simulink model "auv_nmpc_cbf"  (R2024a)
settings: Solver=ode4  StartTime=0.0  StopTime=35  FixedStep=0.010  RelTol=1e-3
values from neighbouring files (symbols this model uses):
  cbfParms = testValues(i,:)    [sweep_auv_cbf.m]
  obstacle = [obs_x , obs_y, obs_z, thisObsRadius]    [sweep_auv_cbf.m]
libraries: simulink x4
settings Model: Creator=mpent  LastModifiedBy=14244039
settings DebuggingCC: UnconnectedInputMsg=warning  UnconnectedOutputMsg=warning  UnconnectedLineMsg=warning
settings ModelReferenceCC: EnableRefExpFcnMdlSchedulingChecks=on
settings RTWCC: GPUComputeCapability=3.5  DLArmComputeVersion=19.05

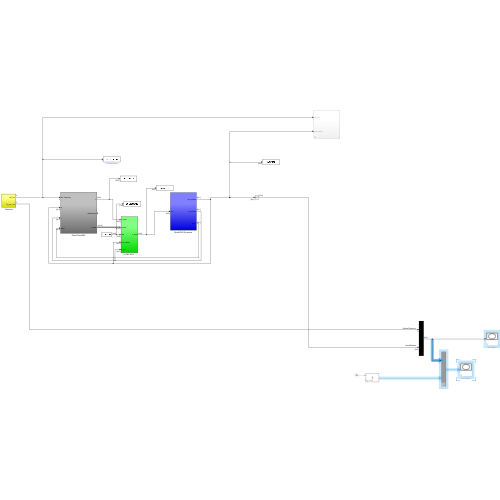
[thumbnail: Simulink's stored preview of the top-level diagram]
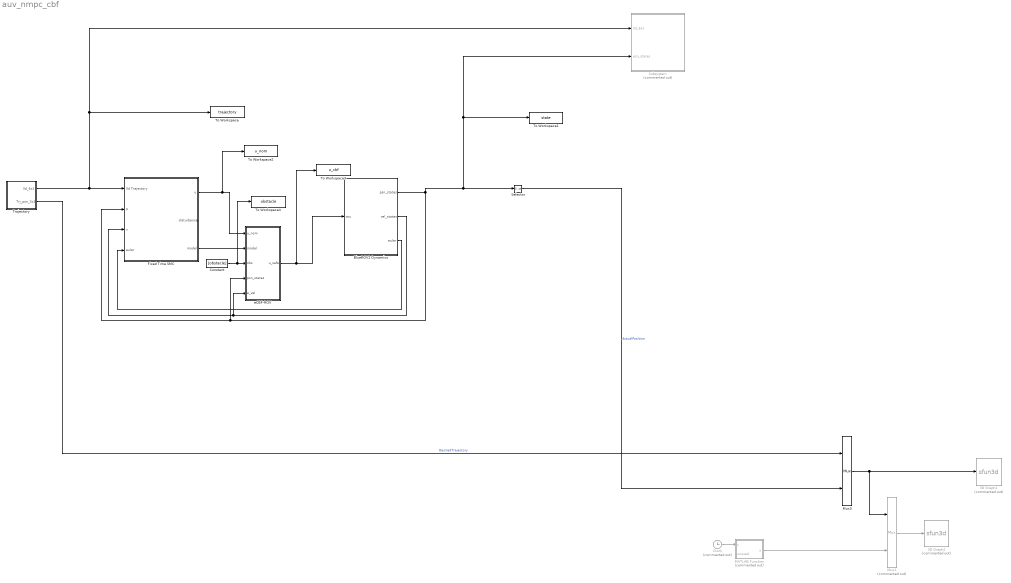
== system auv_nmpc_cbf ==
  3D Graph1 : S-Function  Commented=on  LoadFcn=if exist('sfun3d','file'), sfun3d([],[],[],'LoadBlock'); end  FunctionName=sfun3d  Parameters=ax,T,np,cp,gd,ls,mk,mx,hd,tb  SFunctionDeploymentMode=off  EnableBusSupport=off  mask(3D Graph){np=2, ax=[1 11 1 11 1 11], mx=1e4, T=-1, cp=[180 45 90], gd=on, hd=on, tb=on, ls=-, mk=none}
      mask prompts: np "Number of moving points (lines)"; ax "Range: [xmin xmax  ymin ymax zmin zmax]"; mx "Max number of points in each line"; T "Sampling Time"; cp "Camera position (use [0 0 1] for 2D XY view)"; gd "Grid (on|off)"; hd "HeadMarkers (on|off)"; tb "Toolbar (on|off)"; ls "LineStyle"; mk "LineMarker"
      mask help:
      | This block plots the position of several points in the XYZ space. The input contains the coordinates of all the points (x1,y1,z1,x2,y2,z2,...).
      | The number of moving points (lines), the XYZ ranges, sampling time, camera position, and grid (among other things) can be set as mask parameters.
      settings: CopyFcn=if exist('sfun3d','file'), sfun3d([],[],[],'CopyBlock'); end  DeleteFcn=if exist('sfun3d','file'), sfun3d([],[],[],'DeleteBlock'); end  NameChangeFcn=if exist('sfun3d','file'), sfun3d([],[],[],'NameChange'); end
      mask Help:
      | This block plots the position of several points in the XYZ space. The input contains the coordinates of all the points (x1,y1,z1,x2,y2,z2,...).
      | The number of moving points (lines), the XYZ ranges, sampling time, camera position, and grid (among other things) can be set as mask parameters.
      mask TypeOptions ls: - | -- | : | -. | none
      mask TypeOptions mk: none | . | + | o | * | x | square | diamond | v | ^ | > | < | pentagram | hexagram
      mask Display: plot([.05 .95 .95 .05 .05],[.45 .45 .95 .95 .45], 0.5+cos(0:0.1:2*pi)*0.3,0.7+sin(0:0.1:2*pi)*0.2)
  3D Graph2 : S-Function  Commented=on  LoadFcn=if exist('sfun3d','file'), sfun3d([],[],[],'LoadBlock'); end  FunctionName=sfun3d  Parameters=ax,T,np,cp,gd,ls,mk,mx,hd,tb  SFunctionDeploymentMode=off  EnableBusSupport=off  mask(3D Graph){np=5, ax=[1 11 1 11 1 11], mx=1e4, T=-1, cp=[68.5220  -51.3281   23.4494], gd=on, hd=off, tb=on, ls=-, mk=none}
      mask prompts: np "Number of moving points (lines)"; ax "Range: [xmin xmax  ymin ymax zmin zmax]"; mx "Max number of points in each line"; T "Sampling Time"; cp "Camera position (use [0 0 1] for 2D XY view)"; gd "Grid (on|off)"; hd "HeadMarkers (on|off)"; tb "Toolbar (on|off)"; ls "LineStyle"; mk "LineMarker"
      mask help:
      | This block plots the position of several points in the XYZ space. The input contains the coordinates of all the points (x1,y1,z1,x2,y2,z2,...).
      | The number of moving points (lines), the XYZ ranges, sampling time, camera position, and grid (among other things) can be set as mask parameters.
      settings: CopyFcn=if exist('sfun3d','file'), sfun3d([],[],[],'CopyBlock'); end  DeleteFcn=if exist('sfun3d','file'), sfun3d([],[],[],'DeleteBlock'); end  NameChangeFcn=if exist('sfun3d','file'), sfun3d([],[],[],'NameChange'); end
      mask Help:
      | This block plots the position of several points in the XYZ space. The input contains the coordinates of all the points (x1,y1,z1,x2,y2,z2,...).
      | The number of moving points (lines), the XYZ ranges, sampling time, camera position, and grid (among other things) can be set as mask parameters.
      mask TypeOptions ls: - | -- | : | -. | none
      mask TypeOptions mk: none | . | + | o | * | x | square | diamond | v | ^ | > | < | pentagram | hexagram
      mask Display: plot([.05 .95 .95 .05 .05],[.45 .45 .95 .95 .45], 0.5+cos(0:0.1:2*pi)*0.3,0.7+sin(0:0.1:2*pi)*0.2)
  BlueROV2 Dynamics : Subsystem
  Clock : Clock  Commented=on
  Constant : Constant  Value=[obstacle]  VectorParams1D=off
  Fixed Time SMC : Subsystem
  MATLAB Function : MATLAB Function  Commented=on  TreatAsAtomicUnit=on
  Mux1 : Mux  Commented=on  Inputs=2
  Mux3 : Mux  Inputs=2
  Selector : Selector  InputPortWidth=6  IndexOptions=Index vector (dialog)  Indices=1:3  OutputSizes=1
  Subsystem : Subsystem  Commented=on
  To Workspace : ToWorkspace  VariableName=trajectory  SaveFormat=Timeseries  SampleTime=-1
  To Workspace1 : ToWorkspace  VariableName=state  SaveFormat=Timeseries  SampleTime=-1
  To Workspace2 : ToWorkspace  VariableName=u_nom  SaveFormat=Timeseries  SampleTime=-1
  To Workspace3 : ToWorkspace  VariableName=u_cbf  SaveFormat=Timeseries  SampleTime=-1
  To Workspace4 : ToWorkspace  VariableName=obstacle  SampleTime=-1
      settings: MaxDataPoints=1
  Trajectory : Subsystem
  eCBF-ROV : Subsystem
  wires:
  Mux3/1 -> Mux1/1, 3D Graph1/1
  Selector/1 -> Mux3/2  "ActualPosition"
  Trajectory/2(Trj_psn_3x1) -> Mux3/1  "DesiredTrajectory"
  BlueROV2 Dynamics/2(vel_states) -> Fixed Time SMC/3(v), eCBF-ROV/5(e_vel)
  BlueROV2 Dynamics/1(psn_states) -> To Workspace1/1, Subsystem/2(psn_states), Selector/1, eCBF-ROV/4(psn_states), Fixed Time SMC/2(p)
  BlueROV2 Dynamics/3(euler) -> Fixed Time SMC/4(euler)
  Trajectory/1(Xd_6x1) -> To Workspace/1, Subsystem/1(Xd_6x1), Fixed Time SMC/1(Xd Trajectory)
  Fixed Time SMC/1(u) -> To Workspace2/1, eCBF-ROV/1(u_nom)
  Constant/1 -> To Workspace4/1, eCBF-ROV/3(obs)
  Fixed Time SMC/3(model) -> eCBF-ROV/2(model)
  eCBF-ROV/1(u_safe) -> To Workspace3/1, BlueROV2 Dynamics/1(tau)
  Clock/1 -> MATLAB Function/1(t)
  MATLAB Function/1(y) -> Mux1/2
  Mux1/1 -> 3D Graph2/1

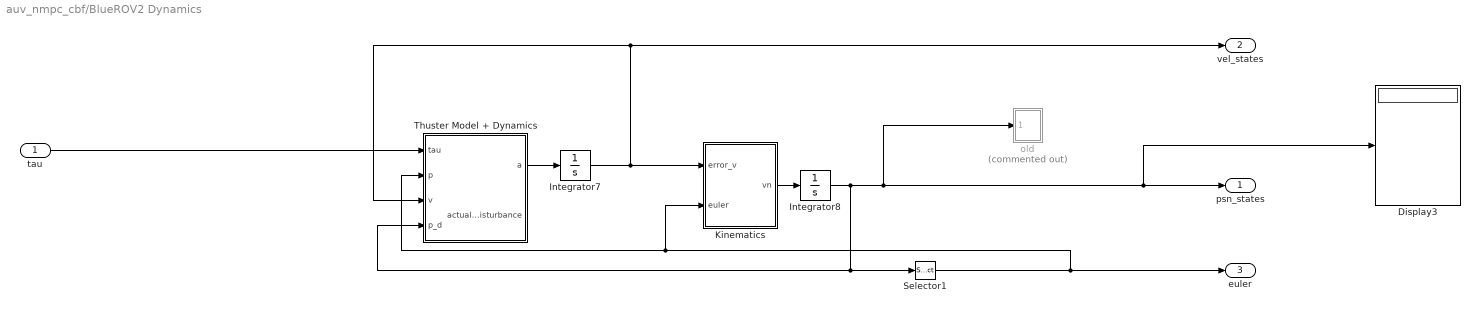
== system auv_nmpc_cbf/BlueROV2 Dynamics ==
  tau : Inport
  Display3 : Display
  Integrator7 : Integrator  InitialCondition=[0 0 0 0 0 0]'  LimitOutput=on  UpperSaturationLimit=[1 1 1 1 1 1]'*2  LowerSaturationLimit=[-1 -1 -1 -1 -1 -1]'*2
  Integrator8 : Integrator  InitialCondition=[1 1 1 0 0 0]'
  Kinematics : MATLAB Function  TreatAsAtomicUnit=on
  Selector1 : Selector  InputPortWidth=6  IndexOptions=Index vector (dialog)  Indices=4:6  OutputSizes=1
  Thuster Model + Dynamics : MATLAB Function  TreatAsAtomicUnit=on
  old : Subsystem  Commented=on
  psn_states : Outport
  vel_states : Outport  Port=2
  euler : Outport  Port=3
  wires:
  Selector1/1 -> Thuster Model + Dynamics/2(p), Kinematics/2(euler), euler/1
  Integrator8/1 -> Selector1/1, Thuster Model + Dynamics/4(p_d), Display3/1, psn_states/1, old/1(In1)
  Thuster Model + Dynamics/1(a) -> Integrator7/1
  Integrator7/1 -> vel_states/1, Thuster Model + Dynamics/3(v), Kinematics/1(error_v)
  tau/1 -> Thuster Model + Dynamics/1(tau)
  Kinematics/1(vn) -> Integrator8/1

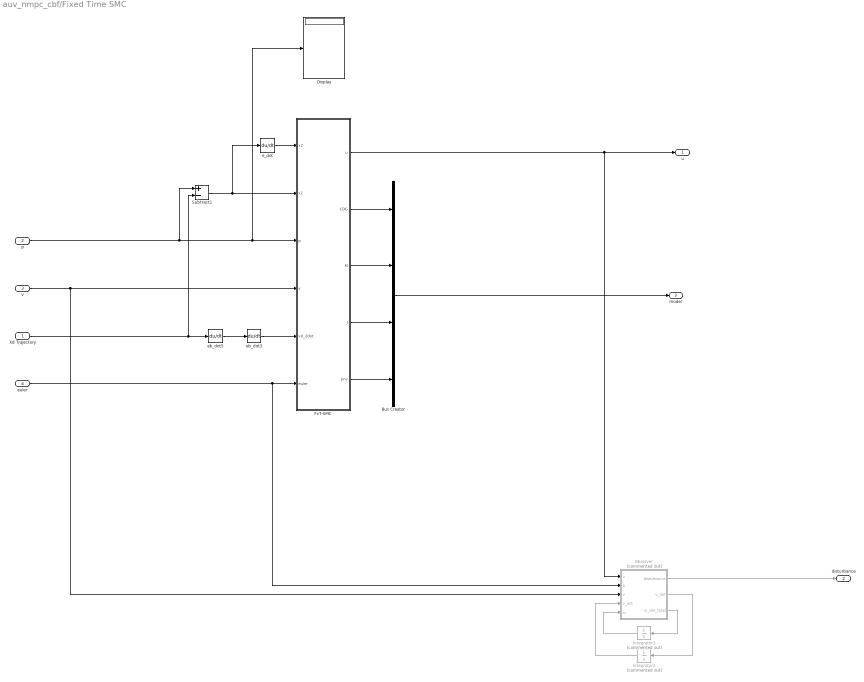
== system auv_nmpc_cbf/Fixed Time SMC ==
  Xd Trajectory : Inport
  p : Inport  Port=2
  v : Inport  Port=3
  euler : Inport  Port=4
  " e_dot" : Derivative
  " eb_dot3" : Derivative
  " eb_dot5" : Derivative
  Bus Creator : BusCreator  Inputs=4
  Display : Display
  FxT-SMC : MATLAB Function  TreatAsAtomicUnit=on
  Integrator2 : Integrator  Commented=on
  Integrator3 : Integrator  Commented=on
  Observer : MATLAB Function  Commented=on  TreatAsAtomicUnit=on
  Subtract1 : Sum  Inputs=+-
  u : Outport
  disturbance : Outport  Port=2
  model : Outport  Port=3
  wires:
  Observer/3(xi_dot_total) -> Integrator3/1
  Subtract1/1 -> " e_dot"/1, FxT-SMC/2(x1)
  " eb_dot3"/1 -> FxT-SMC/5(xd_2dot)
  Observer/2(v_dot) -> Integrator2/1
  FxT-SMC/1(u) -> Observer/1(u), u/1
  euler/1 -> Observer/2(p), FxT-SMC/6(euler)
  " eb_dot5"/1 -> " eb_dot3"/1
  p/1 -> Subtract1/1, Display/1, FxT-SMC/3(p)
  " e_dot"/1 -> FxT-SMC/1(x2)
  Xd Trajectory/1 -> Subtract1/2, " eb_dot5"/1
  v/1 -> Observer/3(v), FxT-SMC/4(v)
  Integrator2/1 -> Observer/4(v_est)
  Integrator3/1 -> Observer/5(xi)
  Observer/1(disturbance) -> disturbance/1
  FxT-SMC/5(Jinv) -> Bus Creator/4
  FxT-SMC/4(J) -> Bus Creator/3
  FxT-SMC/3(M) -> Bus Creator/2
  FxT-SMC/2(CDG) -> Bus Creator/1
  Bus Creator/1 -> model/1

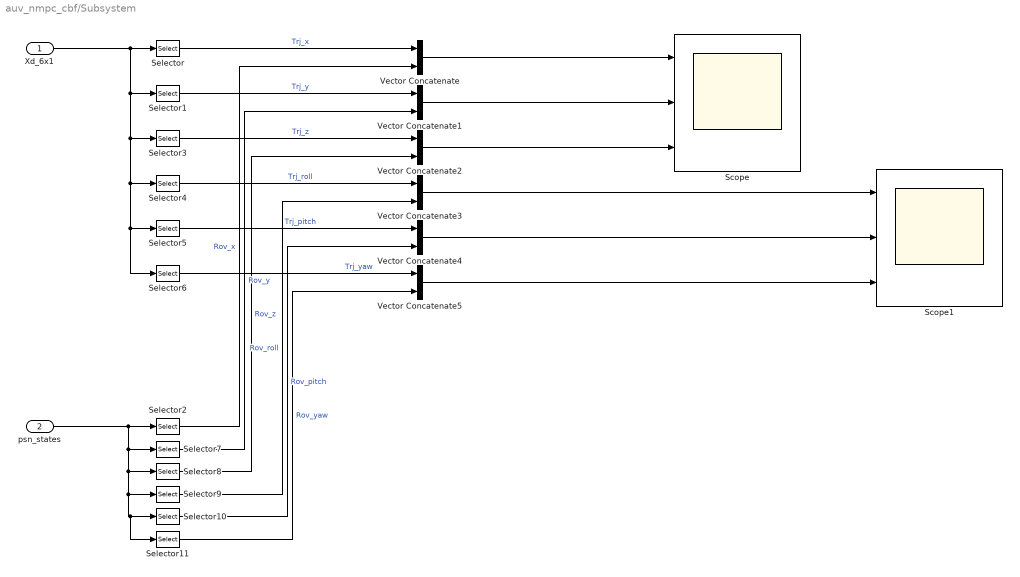
== system auv_nmpc_cbf/Subsystem ==
  Xd_6x1 : Inport
  psn_states : Inport  Port=2
  Scope : Scope  NumInputPorts=3
  Scope1 : Scope  NumInputPorts=3
  Selector : Selector  InputPortWidth=6  IndexOptions=Index vector (dialog)  Indices=1  OutputSizes=1
  Selector1 : Selector  InputPortWidth=6  IndexOptions=Index vector (dialog)  Indices=2  OutputSizes=1
  Selector10 : Selector  InputPortWidth=6  IndexOptions=Index vector (dialog)  Indices=5  OutputSizes=1
  Selector11 : Selector  InputPortWidth=6  IndexOptions=Index vector (dialog)  Indices=6  OutputSizes=1
  Selector2 : Selector  InputPortWidth=6  IndexOptions=Index vector (dialog)  Indices=1  OutputSizes=1
  Selector3 : Selector  InputPortWidth=6  IndexOptions=Index vector (dialog)  Indices=3  OutputSizes=1
  Selector4 : Selector  InputPortWidth=6  IndexOptions=Index vector (dialog)  Indices=4  OutputSizes=1
  Selector5 : Selector  InputPortWidth=6  IndexOptions=Index vector (dialog)  Indices=5  OutputSizes=1
  Selector6 : Selector  InputPortWidth=6  IndexOptions=Index vector (dialog)  Indices=6  OutputSizes=1
  Selector7 : Selector  InputPortWidth=6  IndexOptions=Index vector (dialog)  Indices=2  OutputSizes=1
  Selector8 : Selector  InputPortWidth=6  IndexOptions=Index vector (dialog)  Indices=3  OutputSizes=1
  Selector9 : Selector  InputPortWidth=6  IndexOptions=Index vector (dialog)  Indices=4  OutputSizes=1
  Vector Concatenate{,1..5} (6 alike) : Concatenate
  wires:
  Xd_6x1/1 -> Selector1/1, Selector3/1, Selector4/1, Selector6/1, Selector5/1, Selector/1
  psn_states/1 -> Selector11/1, Selector10/1, Selector9/1, Selector8/1, Selector7/1, Selector2/1
  Selector/1 -> Vector Concatenate/1  "Trj_x"
  Selector2/1 -> Vector Concatenate/2  "Rov_x"
  Selector1/1 -> Vector Concatenate1/1  "Trj_y"
  Selector7/1 -> Vector Concatenate1/2  "Rov_y"
  Selector3/1 -> Vector Concatenate2/1  "Trj_z"
  Selector6/1 -> Vector Concatenate5/1  "Trj_yaw"
  Selector5/1 -> Vector Concatenate4/1  "Trj_pitch"
  Selector4/1 -> Vector Concatenate3/1  "Trj_roll"
  Selector11/1 -> Vector Concatenate5/2  "Rov_yaw"
  Selector10/1 -> Vector Concatenate4/2  "Rov_pitch"
  Selector9/1 -> Vector Concatenate3/2  "Rov_roll"
  Selector8/1 -> Vector Concatenate2/2  "Rov_z"
  Vector Concatenate/1 -> Scope/1
  Vector Concatenate1/1 -> Scope/2
  Vector Concatenate2/1 -> Scope/3
  Vector Concatenate4/1 -> Scope1/2
  Vector Concatenate3/1 -> Scope1/1
  Vector Concatenate5/1 -> Scope1/3

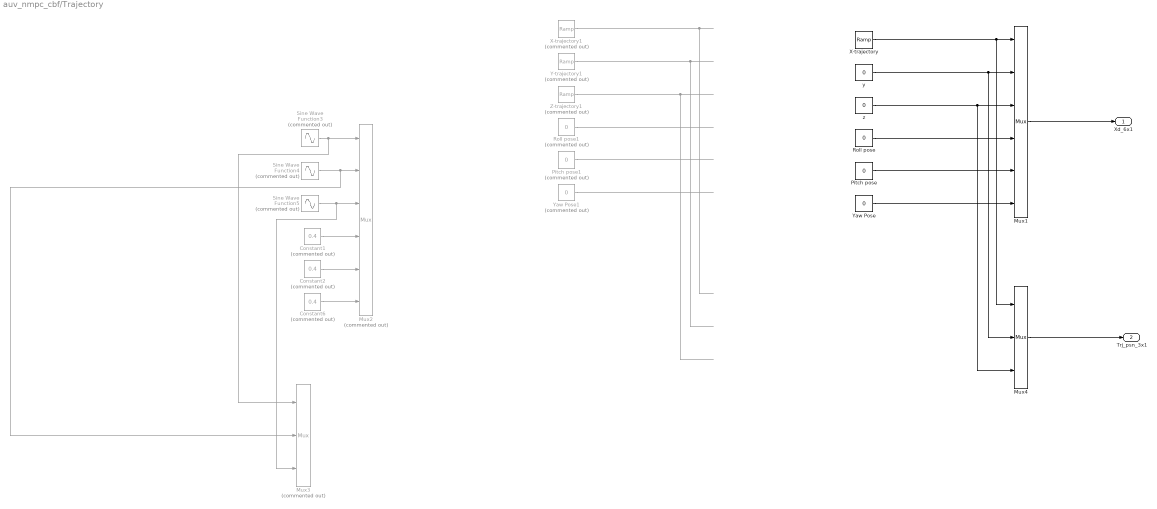
== system auv_nmpc_cbf/Trajectory ==
  Constant1 : Constant  Commented=on  Value=0.4
  Constant2 : Constant  Commented=on  Value=0.4
  Constant6 : Constant  Commented=on  Value=0.4
  Mux1 : Mux  Inputs=6
  Mux2 : Mux  Commented=on  Inputs=6
  Mux3 : Mux  Commented=on  Inputs=3
  Mux4 : Mux  Inputs=3
  Pitch pose : Constant  Value=0
  Pitch pose1 : Constant  Commented=on  Value=0
  Roll pose : Constant  Value=0
  Roll pose1 : Constant  Commented=on  Value=0
  Sine Wave Function3 : Sin  Commented=on  Amplitude=3  Bias=5  Frequency=0.2  SampleTime=0
  Sine Wave Function4 : Sin  Commented=on  Amplitude=4  Bias=5  Frequency=0.3  Phase=pi/2  SampleTime=0
  Sine Wave Function5 : Sin  Commented=on  Amplitude=4  Bias=5  Frequency=0.25  SampleTime=0
  X-trajectory : simulink/Sources/Ramp  slope=1  start=0  InitialOutput=1
  X-trajectory1 : simulink/Sources/Ramp  Commented=on  slope=1  start=0  InitialOutput=1
  Y-trajectory1 : simulink/Sources/Ramp  Commented=on  slope=1  start=0  InitialOutput=1
  Yaw Pose : Constant  Value=0
  Yaw Pose1 : Constant  Commented=on  Value=0
  Z-trajectory1 : simulink/Sources/Ramp  Commented=on  slope=1  start=0  InitialOutput=1
  y : Constant  Value=0
  z : Constant  Value=0
  Xd_6x1 : Outport
  Trj_psn_3x1 : Outport  Port=2
  wires:
  Roll pose/1 -> Mux1/4
  Pitch pose/1 -> Mux1/5
  z/1 -> Mux4/3, Mux1/3
  X-trajectory/1 -> Mux4/1, Mux1/1
  Mux4/1 -> Trj_psn_3x1/1
  y/1 -> Mux4/2, Mux1/2
  Yaw Pose/1 -> Mux1/6
  Mux1/1 -> Xd_6x1/1
  Constant6/1 -> Mux2/6
  Sine Wave Function4/1 -> Mux3/2, Mux2/2
  Sine Wave Function5/1 -> Mux3/3, Mux2/3
  Sine Wave Function3/1 -> Mux3/1, Mux2/1
  Constant1/1 -> Mux2/4
  Constant2/1 -> Mux2/5
  Yaw Pose1/1 -> ?
  Y-trajectory1/1 -> ?
  X-trajectory1/1 -> ?
  Z-trajectory1/1 -> ?
  Pitch pose1/1 -> ?
  Roll pose1/1 -> ?

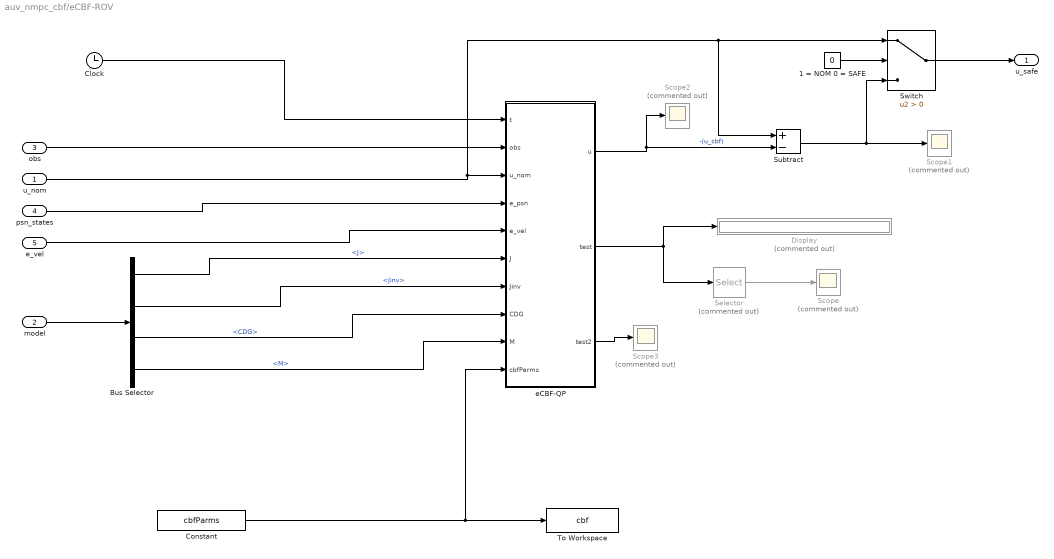
== system auv_nmpc_cbf/eCBF-ROV ==
  u_nom : Inport
  model : Inport  Port=2
  obs : Inport  Port=3
  psn_states : Inport  Port=4
  e_vel : Inport  Port=5
  1 = NOM 0 = SAFE : Constant  Value=0
  Bus Selector : BusSelector  OutputSignals=J,Jinv,CDG,M
  Clock : Clock
  Constant : Constant  Value=cbfParms
  Display : Display  Commented=on
  Scope{,1..3} (4 alike) : Scope  Commented=on
  Selector : Selector  Commented=on  InputPortWidth=4  IndexOptions=Index vector (dialog)  Indices=4  OutputSizes=1
  Subtract : Sum  Inputs=+-
  Switch : Switch  Criteria=u2 > Threshold  SaturateOnIntegerOverflow=off  InputSameDT=off
  To Workspace : ToWorkspace  VariableName=cbf  SampleTime=-1
      settings: MaxDataPoints=1
  eCBF-QP : MATLAB Function  TreatAsAtomicUnit=on
  u_safe : Outport
  wires:
  u_nom/1 -> Subtract/1, Switch/1, eCBF-QP/3(u_nom)
  model/1 -> Bus Selector/1
  Bus Selector/3 -> eCBF-QP/8(CDG)  "<CDG>"
  Bus Selector/4 -> eCBF-QP/9(M)  "<M>"
  Bus Selector/1 -> eCBF-QP/6(J)  "<J>"
  Bus Selector/2 -> eCBF-QP/7(Jinv)  "<Jinv>"
  obs/1 -> eCBF-QP/2(obs)
  psn_states/1 -> eCBF-QP/4(e_psn)
  e_vel/1 -> eCBF-QP/5(e_vel)
  eCBF-QP/2(test) -> Display/1, Selector/1
  Selector/1 -> Scope/1
  Clock/1 -> eCBF-QP/1(t)
  eCBF-QP/1(u) -> Scope2/1, Subtract/2  "-(u_cbf)"
  Subtract/1 -> Switch/3, Scope1/1
  1 = NOM 0 = SAFE/1 -> Switch/2
  Switch/1 -> u_safe/1
  eCBF-QP/3(test2) -> Scope3/1
  Constant/1 -> eCBF-QP/10(cbfParms), To Workspace/1

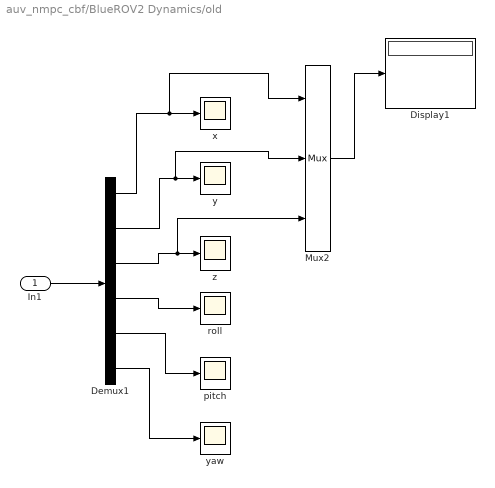
== system auv_nmpc_cbf/BlueROV2 Dynamics/old ==
  In1 : Inport
  Demux1 : Demux  Outputs=6
  Display1 : Display
  Mux2 : Mux  Inputs=3
  pitch : Scope
  roll : Scope
  x : Scope
  y : Scope
  yaw : Scope
  z : Scope
  wires:
  Demux1/3 -> Mux2/3, z/1
  Demux1/1 -> Mux2/1, x/1
  Demux1/4 -> roll/1
  Demux1/5 -> pitch/1
  Demux1/2 -> Mux2/2, y/1
  In1/1 -> Demux1/1
  Demux1/6 -> yaw/1
  Mux2/1 -> Display1/1

== matlab function auv_nmpc_cbf/Fixed Time SMC/Observer ==
  data: disturbance output size=[6 1]; u input; p input; v_dot output size=[6 1]; v input; v_est input; xi input; xi_dot_total output size=[6 1]
function [disturbance, v_dot, xi_dot_total]= fcn(u, p, v, v_est, xi)

%% Declaring variables
m=11.5;
W=112.8;
B=114.8;

Ix=0.16;
Iy=0.16;
Iz=0.16;

Xu_d = -5.5;
Yv_d = -12.7;
Zw_d = -14.57;
Kp_d = -0.12;
Mq_d = -0.12;
Nr_d = -0.12;

Xu = -4.03;
Yv = -6.22;
Zw = -5.18;
Kp = -0.07;
Mq = -0.07;
Nr = -0.07;

Xuu = -18.18;
Yvv = -21.66;
Zww = -36.99;
Kpp = -1.55;
Mqq = -1.55;
Nrr = -1.55;

rb = [0; 0; 0];
rg = [0; 0; 0.02];

%% Mass Matrix - Mrb + Ma
M_total = [m-Xu_d        0        0         0      m*rg(3)      0;
             0        m-Yv_d      0      -m*rg(3)   0           0;   
             0          0      m-Zw_d       0       0           0;
             0        -m*rg(3)    0      Ix-Kp_d    0           0;
           m*rg(3)      0         0         0     Iy-Mq_d       0;
             0          0         0         0       0        Iz-Nr_d;];



%% Coriolis and Centripetal Matrix - Crb + Ca
C_total = [v(5)*(Zw_d*v(3) + m*v(3));
           - v(4)*(Zw_d*v(3) + m*v(3)) - Xu_d*v(1)*v(6);
           v(5)*(Xu_d*v(1) - m*v(1)) - v(4)*(Yv_d*v(2) - m*v(2));
v(5)*(Iz*v(6) - Nr_d*v(6)) - v(6)*(Iy*v(5) - Mq_d*v(5)) + v(3)*(Yv_d*v(2) - m*v(2)) - v(2)*(Zw_d*v(3) - m*v(3));
v(6)*(Ix*v(4) - Kp_d*v(4)) - v(4)*(Iz*v(6) - Nr_d*v(6)) - v(3)*(Xu_d*v(1) + m*v(1)) + v(1)*(Zw_d*v(3) - m*v(3));
v(4)*(Iy*v(5) - Mq_d*v(5)) - v(5)*(Ix*v(4) - Kp_d*v(4)) + v(2)*(Xu_d*v(1) - m*v(1)) - v(1)*(Yv_d*v(2) - m*v(2));];

%% Hydrodynamic Damping
D = -[(Xu+(Xuu*abs(v(1))))*v(1);
       (Yv+(Yvv*abs(v(2))))*v(2);
       (Zw+(Zww*abs(v(3))))*v(3);
       (Kp+(Kpp*abs(v(4))))*v(4);
       (Mq+(Mqq*abs(v(5))))*v(5);
       (Nr+(Nrr*abs(v(6))))*v(6);];

%% Restoring Forces 
g = [      (W-B)*sin(p(2));
        -(W-B)*cos(p(2))*sin(p(1));
        -(W-B)*cos(p(2))*cos(p(1));
        rg(3)*W*cos(p(2))*sin(p(1));
            rg(3)*W*sin(p(2));
                    0;];

%% Declaring variables for observer

rho = 5;
epsilon = 0.5;
K1 = 10;
K2 = 20;
gamma1 = 0.5;
gamma2 = 2.5;
e = v - v_est;  %v_est = integral of v_dot

Kt = 5;
mu = 10; 

%% Calculate xi_dot
xi_dot1 = Kt*sign(e(1));
xi_dot2 = Kt*sign(e(2));
xi_dot3 = Kt*sign(e(3));
xi_dot4 = Kt*sign(e(4));
xi_dot5 = Kt*sign(e(5));
xi_dot6 = Kt*sign(e(6));

xi_dot_total = [xi_dot1;
            xi_dot2;
            xi_dot3;
            xi_dot4;
            xi_dot5;
            xi_dot6;];

%% Calculate ustw
ustw1 = mu*(abs(e(1))^(0.5))*sign(e(1)) + xi(1);
ustw2 = mu*(abs(e(2))^(0.5))*sign(e(2)) + xi(2);
ustw3 = mu*(abs(e(3))^(0.5))*sign(e(3)) + xi(3);
ustw4 = mu*(abs(e(4))^(0.5))*sign(e(4)) + xi(4);
ustw5 = mu*(abs(e(5))^(0.5))*sign(e(5)) + xi(5);
ustw6 = mu*(abs(e(6))^(0.5))*sign(e(6)) + xi(6);

ustw_total = [ustw1;
              ustw2;
              ustw3;
              ustw4;
              ustw5;
              ustw6;];

%%

omega1 = ustw1 + K1*(abs(e(1))^gamma1)*sign(e(1)) + K2*(abs(e(1))^gamma2)*sign(e(1));
omega2 = ustw2 + K1*(abs(e(2))^gamma1)*sign(e(2)) + K2*(abs(e(2))^gamma2)*sign(e(2));
omega3 = ustw3 + K1*(abs(e(3))^gamma1)*sign(e(3)) + K2*(abs(e(3))^gamma2)*sign(e(3));
omega4 = ustw4 + K1*(abs(e(4))^gamma1)*sign(e(4)) + K2*(abs(e(4))^gamma2)*sign(e(4));
omega5 = ustw5 + K1*(abs(e(5))^gamma1)*sign(e(5)) + K2*(abs(e(5))^gamma2)*sign(e(5));
omega6 = ustw6 + K1*(abs(e(6))^gamma1)*sign(e(6)) + K2*(abs(e(6))^gamma2)*sign(e(6));

omega = [omega1;
         omega2;
         omega3;
         omega4;
         omega5;
         omega6;];

%% Output
v_dot = inv(M_total)*(u - C_total - D - g) + omega;

%% Output - disturbance observed
disturbance = ustw_total;

== matlab function auv_nmpc_cbf/MATLAB Function ==
  data: t input; y output; unused input
function y = fcn(t,~)
    center = [5 ; 5 ; 5];
    radius = 0.5;
    theta = t*10*(2*pi/10)-(pi/2);
    traj1 = center + radius*[   0*ones(size(theta));    cos(theta);             sin(theta)              ];
    traj2 = center + radius*[   sin(theta);             0*ones(size(theta));    cos(theta)              ];
    traj3 = center + radius*[   cos(theta);             sin(theta);             0*ones(size(theta))     ];

       
    y = [traj1; traj2; traj3];

== matlab function auv_nmpc_cbf/eCBF-ROV/eCBF-QP ==
  settings: updateMethod=DISCRETE
  data: t input; obs input; u_nom input; e_psn input; e_vel input; u output; J input; Jinv input; CDG input; test output; test2 output; M input; cbfParms input
function [u, test, test2]       = fcn(t,obs,u_nom,e_psn,e_vel,J,Jinv,CDG,M, cbfParms)
%% debug - mute output first few timesteps
    if t < 0.005;
        mute    =0;
    else
        mute    =1;
    end
%% Parameters
    tstep   = 0.001;


%% Persistent Variables
    persistent Jprev;

    if isempty(Jprev)
        Jprev = J;
    end

%% Derivative Variables

    Jdot = (J - Jprev)/ tstep;
    Jprev = J;

%% System states from inputs

        % Variables used in ECBF
        m           = inv(M);
        k1          = cbfParms(1);
        k2          = cbfParms(2);
        rpad        = 0.5;     % additional clearance to obstacle

        
        %earth frame positions
        pos_x       = e_psn(1);
        pos_y       = e_psn(2);
        pos_z     	= e_psn(3);
        roll        = e_psn(4);
        pitch       = e_psn(5);
        yaw         = e_psn(6);
                
        %earth frame velocities [eta_dot]        
        earth_v     = 1*e_vel;    % transform velocities to earth frame from rov frame
        
        e_vel_x     = earth_v(1);
        e_vel_y     = earth_v(2);
        e_vel_z     = earth_v(3);
        
        %earth frame accelerations [eta_dot_dot]
        ctrl        = u_nom;
        earth_acc   = J*m*(ctrl - CDG) + Jdot*(Jinv*e_vel);
        
        e_acc_x     = earth_acc(1);
        e_acc_y     = earth_acc(2);
        e_acc_z     = earth_acc(3);

       
        % Obstacle parameters
        r_obs       = obs(4);
        obs_x       = obs(1);
        obs_y       = obs(2);
        obs_z       = obs(3);
        
        a           = 2*r_obs;      % for circular obstacle
        b           = a;            % for circular obstacle
        c           = a;
        
        sep_x       = pos_x - obs_x;
        sep_y       = pos_y - obs_y;
        sep_z       = pos_z - obs_z;
        
        SEP         = [2*a*sep_x ; 2*b*sep_y ; 2*c*sep_z ; 0 ; 0 ; 0]';
%         S           = [2*a*Sx   2*b*Sy  ];
%         S2          = [2*a*S2x  2*b*S2y ]; 
        
%%    Barrier function 
        h           = a*( sep_x^2 ) + ...
                      b*( sep_y^2 ) + ...
                      c*( sep_z^2 ) - rpad ;
        
        Lfh         = 2*a*(sep_x)*(e_vel_x) +...
                      2*b*(sep_y)*(e_vel_y) +...
                      2*c*(sep_z)*(e_vel_z);
             
%         L2fh        = 2*a*(sep_x)*e_acc_x + 2*a*(e_vel_x^2) +...
%                       2*b*(sep_y)*e_acc_y + 2*a*(e_vel_y^2) +...
%                       2*c*(sep_z)*e_acc_z + 2*c*(e_vel_z^2)     ;
                  
%        ECBF        = L2fh*mute + k1*Lfh*mute + k2*h;

    % quadprog parameters
 
    H       = 2*[   1 0 0 0 0 0 ; ...
                    0 1 0 0 0 0 ; ... 
                    0 0 1 0 0 0 ; ...
                    0 0 0 1 0 0 ; ...
                    0 0 0 0 1 0 ; ...
                    0 0 0 0 0 1 ];
        
    f       = [0;0;0;0;0;0]; 
    
    % Setup A & b matrices
        A       =  SEP * (J * m) ;
        b       =  SEP * (J * m*(ctrl - CDG) + Jdot*e_vel) ... 
                    + 2*a*e_vel_x^2 + 2*b*e_vel_y^2 + 2*c*e_vel_z ...
                    + k1*Lfh  + k2*h       ;

    u_qp   = [0;0;0;0;0;0];
    flag = 0;
    coder.extrinsic('quadprog');
    options = optimset('Display','off');
    [output, ~, flag]   = quadprog(H,f,A,b,[],[],[],[],[],options);

    if flag == 1
        u_qp = output;
    else
        u_qp   = [0;0;0;0;0;0];
    end
    %}
%% Function outputs
    test    = [h Lfh 0 0];
    test2   = flag;
    u       = u_qp;

== matlab function auv_nmpc_cbf/Fixed Time SMC/FxT-SMC ==
  data: x2 input; x1 input; p input; v input; xd_2dot input size=[6 1]; u output size=[6 1]; euler input size=[3 1]; CDG output; M output; J output; Jinv output
function [u, CDG, M, J, Jinv] = fcn(x2, x1, p, v, xd_2dot, euler)

%% Declaring variables

m=11.5;
W=112.8;
B=114.8;

Ix=0.16;
Iy=0.16;
Iz=0.16;

Xu_d = -5.5;
Yv_d = -12.7;
Zw_d = -14.57;
Kp_d = -0.12;
Mq_d = -0.12;
Nr_d = -0.12;

Xu = -4.03;
Yv = -6.22;
Zw = -5.18;
Kp = -0.07;
Mq = -0.07;
Nr = -0.07;

Xuu = -18.18;
Yvv = -21.66;
Zww = -36.99;
Kpp = -1.55;
Mqq = -1.55;
Nrr = -1.55;

rb = [0; 0; 0];
rg = [0; 0; 0.02];

%% Mass Matrix - Mrb + Ma
M_total = [m-Xu_d        0        0         0      m*rg(3)      0;
             0        m-Yv_d      0      -m*rg(3)   0           0;   
             0          0      m-Zw_d       0       0           0;
             0        -m*rg(3)    0      Ix-Kp_d    0           0;
           m*rg(3)      0         0         0     Iy-Mq_d       0;
             0          0         0         0       0        Iz-Nr_d;];



%% Coriolis and Centripetal Matrix - Crb + Ca
C_total = [v(5)*(Zw_d*v(3) + m*v(3));
           - v(4)*(Zw_d*v(3) + m*v(3)) - Xu_d*v(1)*v(6);
           v(5)*(Xu_d*v(1) - m*v(1)) - v(4)*(Yv_d*v(2) - m*v(2));
v(5)*(Iz*v(6) - Nr_d*v(6)) - v(6)*(Iy*v(5) - Mq_d*v(5)) + v(3)*(Yv_d*v(2) - m*v(2)) - v(2)*(Zw_d*v(3) - m*v(3));
v(6)*(Ix*v(4) - Kp_d*v(4)) - v(4)*(Iz*v(6) - Nr_d*v(6)) - v(3)*(Xu_d*v(1) + m*v(1)) + v(1)*(Zw_d*v(3) - m*v(3));
v(4)*(Iy*v(5) - Mq_d*v(5)) - v(5)*(Ix*v(4) - Kp_d*v(4)) + v(2)*(Xu_d*v(1) - m*v(1)) - v(1)*(Yv_d*v(2) - m*v(2));];

%% Hydrodynamic Damping
D = -[(Xu+(Xuu*abs(v(1))))*v(1);
       (Yv+(Yvv*abs(v(2))))*v(2);
       (Zw+(Zww*abs(v(3))))*v(3);
       (Kp+(Kpp*abs(v(4))))*v(4);
       (Mq+(Mqq*abs(v(5))))*v(5);
       (Nr+(Nrr*abs(v(6))))*v(6);];

%% Restoring Forces 
g = [      (W-B)*sin(p(5));
        -(W-B)*cos(p(5))*sin(p(4));
        -(W-B)*cos(p(5))*cos(p(4));
        rg(3)*W*cos(p(5))*sin(p(4));
            rg(3)*W*sin(p(5));
                    0;];

%% Jacobian Matrix - transform body-fixed frame to earth-fixed frame
J_n = [cos(euler(3))*cos(euler(2)),            cos(euler(3))*sin(euler(1))*sin(euler(2)) - cos(euler(1))*sin(euler(3)),         sin(euler(1))*sin(euler(3)) + cos(euler(1))*cos(euler(3))*sin(euler(2)),                              0                                                0                                                                0        ;
    cos(euler(2))*sin(euler(3)),              cos(euler(1))*cos(euler(3)) + sin(euler(1))*sin(euler(3))*sin(euler(2)),          cos(euler(1))*sin(euler(3))*sin(euler(2)) - cos(euler(3))*sin(euler(1)),                              0                                                0                                                                0        ;
    -sin(euler(2)),                              cos(euler(2))*sin(euler(1)),                                             cos(euler(1))*cos(euler(2))                                              0                                                0                                                                0        ;
    0                                                0                                                                0,                                                        1,                            sin(euler(1))*tan(euler(2))                            cos(euler(1))*tan(euler(2));
    0                                                0                                                                0,                                                        0,                                            cos(euler(1)),                                           -sin(euler(1))                ;
    0                                                0                                                                0,                                                        0,                                 sin(euler(1))/cos(euler(2)),                                                 cos(euler(1))/cos(euler(2));];

%% Inverse Jacobian Matrix - transform body-fixed frame to earth-fixed frame
J_inverse = [ cos(euler(3))*cos(euler(2)),                                  cos(euler(2))*sin(euler(3)),                                      -sin(euler(2)),                               0,                 0,                0;
    cos(euler(3))*sin(euler(1))*sin(euler(2)) - cos(euler(1))*sin(euler(3)),      cos(euler(1))*cos(euler(3)) + sin(euler(1))*sin(euler(3))*sin(euler(2)),     cos(euler(2))*sin(euler(1)),                   0,                 0,                 0;
    sin(euler(1))*sin(euler(3)) + cos(euler(1))*cos(euler(3))*sin(euler(2)),      cos(euler(1))*sin(euler(3))*sin(euler(2)) - cos(euler(3))*sin(euler(1)),             cos(euler(1))*cos(euler(2)),          0,                 0,                 0;
                0,                                                          0,                                                  0,                      1,                   0,        -sin(euler(2));
                0,                                                          0,                                                  0,                       0,             cos(euler(1)),         cos(euler(2))*sin(euler(1));
                0,                                                          0,                                                  0,                       0,             -sin(euler(1)),        cos(euler(2))*cos(euler(1))];


%% Declaring variables used in Fixed-Time SMC
K1 = 5;
K2 = 5;
alpha = 0.5;
gamma = 1.2;
K = 5;
lambda1 = 5;
lambda2 = 5;
m1 = 0.5;
m2 = 1.2;

%% S
s1 = x2(1) + K1*((abs(x1(1))^alpha)*sign(x1(1))) + K2*((abs(x1(1))^gamma)*sign(x1(1)));
s2 = x2(2) + K1*((abs(x1(2))^alpha)*sign(x1(2))) + K2*((abs(x1(2))^gamma)*sign(x1(2)));
s3 = x2(3) + K1*((abs(x1(3))^alpha)*sign(x1(3))) + K2*((abs(x1(3))^gamma)*sign(x1(3)));
s4 = x2(4) + K1*((abs(x1(4))^alpha)*sign(x1(4))) + K2*((abs(x1(4))^gamma)*sign(x1(4)));
s5 = x2(5) + K1*((abs(x1(5))^alpha)*sign(x1(5))) + K2*((abs(x1(5))^gamma)*sign(x1(5)));
s6 = x2(6) + K1*((abs(x1(6))^alpha)*sign(x1(6))) + K2*((abs(x1(6))^gamma)*sign(x1(6)));

%% ueq

omega1 = xd_2dot(1) - K1*alpha*((abs(x1(1))^(alpha-1))*x2(1)) - K2*gamma*((abs(x1(1))^(gamma-1))*x2(1));
omega2 = xd_2dot(2) - K1*alpha*((abs(x1(2))^(alpha-1))*x2(2)) - K2*gamma*((abs(x1(2))^(gamma-1))*x2(2));
omega3 = xd_2dot(3) - K1*alpha*((abs(x1(3))^(alpha-1))*x2(3)) - K2*gamma*((abs(x1(3))^(gamma-1))*x2(3));
omega4 = xd_2dot(4) - K1*alpha*((abs(x1(4))^(alpha-1))*x2(4)) - K2*gamma*((abs(x1(4))^(gamma-1))*x2(4));
omega5 = xd_2dot(5) - K1*alpha*((abs(x1(5))^(alpha-1))*x2(5)) - K2*gamma*((abs(x1(5))^(gamma-1))*x2(5));
omega6 = xd_2dot(6) - K1*alpha*((abs(x1(6))^(alpha-1))*x2(6)) - K2*gamma*((abs(x1(6))^(gamma-1))*x2(6));

omega_total = [omega1;
               omega2;
               omega3;
               omega4;
               omega5;
               omega6;];
           
for i = 1:6                         %%temp fix for initial nan values
    if isnan(omega_total(i))
        omega_total(i) = 0;
    end
end


ueq_total = J_inverse*M_total*omega_total + C_total + D + g - M_total*J_n*v;


%% us
beta1 = -K*sign(s1) - lambda1*((abs(s1)^m1)*sign(s1)) - lambda2*((abs(s1)^m2)*sign(s1));
beta2 = -K*sign(s2) - lambda1*((abs(s2)^m1)*sign(s2)) - lambda2*((abs(s2)^m2)*sign(s2));
beta3 = -K*sign(s3) - lambda1*((abs(s3)^m1)*sign(s3)) - lambda2*((abs(s3)^m2)*sign(s3));
beta4 = -K*sign(s4) - lambda1*((abs(s4)^m1)*sign(s4)) - lambda2*((abs(s4)^m2)*sign(s4));
beta5 = -K*sign(s5) - lambda1*((abs(s5)^m1)*sign(s5)) - lambda2*((abs(s5)^m2)*sign(s5));
beta6 = -K*sign(s6) - lambda1*((abs(s6)^m1)*sign(s6)) - lambda2*((abs(s6)^m2)*sign(s6));

beta_total = [beta1;
              beta2;
              beta3;
              beta4;
              beta5;
              beta6;];

us_total = M_total*(beta_total);


%% u = ueq + us
u_total = ueq_total + us_total;



%% Control Allocation as BlueROV2 has 8 thrusters but 6 DoF (Over Acuatated)

% Thruster Configuration Matrix
T = [0.707 0.707 -0.707 -0.707 0 0 0 0;
    -0.707 0.707 -0.707 0.707 0 0 0 0;
    0 0 0 0 -1 1 1 -1;
    0.06 -0.06 0.06 -0.06 -0.218 -0.218 0.218 0.218;
    0.06 0.06 -0.06 -0.06 0.120 -0.120 0.120 -0.120;
    -0.1888 0.1888 0.1888 -0.1888 0 0 0 0;];

% Thruster Coefficient
K = [40 0 0 0 0 0 0 0;
    0 40 0 0 0 0 0 0;
    0 0 40 0 0 0 0 0;
    0 0 0 40 0 0 0 0;
    0 0 0 0 40 0 0 0;
    0 0 0 0 0 40 0 0;
    0 0 0 0 0 0 40 0;
    0 0 0 0 0 0 0 40;];


% Control Allocation
u_alloc = inv(K)*pinv(T)*u_total;

% Generalised input control to dynamics block
u = T*K*u_alloc;


%Added outputs
CDG = C_total + D + g;

M = M_total;

J = J_n;

Jinv = J_inverse;

== matlab function auv_nmpc_cbf/BlueROV2 Dynamics/Kinematics ==
  data: error_v input; euler input; vn output size=[6 1]
function vn= fcn(error_v, euler)

%% Euler transformation of velocity in the body-fixed frame to velocity in the earth-fixed frame
J_n = [ cos(euler(3))*cos(euler(2)),    cos(euler(3))*sin(euler(1))*sin(euler(2)) - cos(euler(1))*sin(euler(3)),    sin(euler(1))*sin(euler(3)) + cos(euler(1))*cos(euler(3))*sin(euler(2)),    0,      0,                              0                           ;
        cos(euler(2))*sin(euler(3)),    cos(euler(1))*cos(euler(3)) + sin(euler(1))*sin(euler(3))*sin(euler(2)),    cos(euler(1))*sin(euler(3))*sin(euler(2)) - cos(euler(3))*sin(euler(1)),    0,      0,                              0                           ;
        -sin(euler(2)),                 cos(euler(2))*sin(euler(1)),                                                cos(euler(1))*cos(euler(2))                                                 0,      0,                              0                           ;
        0,                              0,                                                                           0,                                                                         1,      sin(euler(1))*tan(euler(2)),    cos(euler(1))*tan(euler(2)) ;
        0,                              0,                                                                           0,                                                                         0,      cos(euler(1)),                  -sin(euler(1))              ;
        0,                              0,                                                                           0,                                                                         0,      sin(euler(1))/cos(euler(2)),    cos(euler(1))/cos(euler(2)) ;   ];

%% Output - Earth-fixed Velocity
vn = J_n*error_v;

== matlab function auv_nmpc_cbf/BlueROV2 Dynamics/Thuster Model + Dynamics ==
  data: tau input; p input; a output size=[6 1]; v input; actual_disturbance output size=[6 1]; p_d input
function [a, actual_disturbance]= fcn(tau, p, v, p_d)
%% Declaring variables

    m       =11.5;
    W       =112.8;
    B       =114.8;

    Ix      =0.16;
    Iy      =0.16;
    Iz      =0.16;

    Xu_d    = -5.5;
    Yv_d    = -12.7;
    Zw_d    = -14.57;
    Kp_d    = -0.12;
    Mq_d    = -0.12;
    Nr_d    = -0.12;

    Xu      = -4.03;
    Yv      = -6.22;
    Zw      = -5.18;
    Kp      = -0.07;
    Mq      = -0.07;
    Nr      = -0.07;

    Xuu     = -18.18;
    Yvv     = -21.66;
    Zww     = -36.99;
    Kpp     = -1.55;
    Mqq     = -1.55;
    Nrr     = -1.55;

    rb      = [0; 0; 0];
    rg      = [0; 0; 0.02];

%% Mass Matrix - Mrb + Ma
M_total = [     m-Xu_d      0           0           0           m*rg(3)         0;
                0           m-Yv_d      0           -m*rg(3)    0               0;   
                0           0           m-Zw_d      0           0               0;
                0           -m*rg(3)    0           Ix-Kp_d     0               0;
                m*rg(3)     0           0           0           Iy-Mq_d         0;
                0           0           0           0           0               Iz-Nr_d;   ];



%% Coriolis and Centripetal Matrix - Crb + Ca
C_total = [     v(5)*(Zw_d*v(3) + m*v(3));
                -v(4)*(Zw_d*v(3) + m*v(3)) - Xu_d*v(1)*v(6);
                v(5)*(Xu_d*v(1) - m*v(1)) - v(4)*(Yv_d*v(2) - m*v(2));
                v(5)*(Iz*v(6) - Nr_d*v(6)) - v(6)*(Iy*v(5) - Mq_d*v(5)) + v(3)*(Yv_d*v(2) - m*v(2)) - v(2)*(Zw_d*v(3) - m*v(3));
                v(6)*(Ix*v(4) - Kp_d*v(4)) - v(4)*(Iz*v(6) - Nr_d*v(6)) - v(3)*(Xu_d*v(1) + m*v(1)) + v(1)*(Zw_d*v(3) - m*v(3));
                v(4)*(Iy*v(5) - Mq_d*v(5)) - v(5)*(Ix*v(4) - Kp_d*v(4)) + v(2)*(Xu_d*v(1) - m*v(1)) - v(1)*(Yv_d*v(2) - m*v(2));  ];

%% Hydrodynamic Damping
D = -[  (Xu+(Xuu*abs(v(1))))*v(1);
        (Yv+(Yvv*abs(v(2))))*v(2);
        (Zw+(Zww*abs(v(3))))*v(3);
        (Kp+(Kpp*abs(v(4))))*v(4);
        (Mq+(Mqq*abs(v(5))))*v(5);
        (Nr+(Nrr*abs(v(6))))*v(6);  ];

%% Restoring Forces 
g = [   (W-B)*sin(p(2));
        -(W-B)*cos(p(2))*sin(p(1));
        -(W-B)*cos(p(2))*cos(p(1));
        rg(3)*W*cos(p(2))*sin(p(1));
        rg(3)*W*sin(p(2));
        0;                              ];

%% Addition of disturbance matrix for disturbance observer
disturbance = [0;
               0;
               0;
               0;
               0;
               0;       ];

%{
% disturbance = [ 1.5*v(1) + sin(3*p_d(1)) + 1.5*sin(v(1));
%                 1.5*v(2) - 2*sin(2*p_d(1)) + 1.3*sin(v(2));
%                 -1.2*v(3) - 2*sin(p_d(3)) + 1.13*sin(v(3));
%                 1.5*v(4) + sin(3*p_d(4)) + 1.5*sin(v(4));
%                 1.5*v(5) - 2*sin(2*p_d(4)) + 1.3*sin(v(5));
%                 -1.2*v(6) - 2*sin(p_d(6)) + 1.13*sin(v(6));];


% disturbance = [ -5*v(1)^2 - 7*sin(v(1)*v(2));
%                6.1*v(1)^2 + 7.5*sin(v(2));
%                  7*v(1)^2 + 8*sin(v(3));
%                  2*v(4)^3;
%                  -2*v(5)^2;
%                  -3.2*v(6)^3;];
%}

%% Output - Acceleration
a = inv(M_total)*(tau - C_total - D - g - disturbance);

%% Output - Actual Disturbance (feeds into observer block)
actual_disturbance = zeros(6,1); % ### remove this for now ### % inv(M_total)*(-disturbance);
